simulink model "PT1sys"  (R2016b)
settings: Solver=VariableStepAuto  StartTime=0.0  StopTime=15  RelTol=1e-3
values from neighbouring files (symbols this model uses):
  r1 = 0.0191    [LQG.m]    (also in RiccatiBerechnung_Anlage.m = 0.046; RiccatiBerechnunguPlot_Simulation.m = 0.046; StartSim.m = 0.046)
  T1 = 0.1    [LQG.m]    (also in RiccatiBerechnung_Anlage.m = 0.03032; RiccatiBerechnunguPlot_Simulation.m = 0.03032; StartSim.m = 0.03032)
  T2 = 0.1    [LQG.m]    (also in RiccatiBerechnung_Anlage.m = 0.0247; RiccatiBerechnunguPlot_Simulation.m = 0.0247; StartSim.m = 0.03032)
undefined symbols (not defined in the file or in its folder): K, k1, k2, n01, n02
libraries: simulink x4, simulink_extras x2
settings Model: Creator=Patrick  LastModifiedBy=Patrick

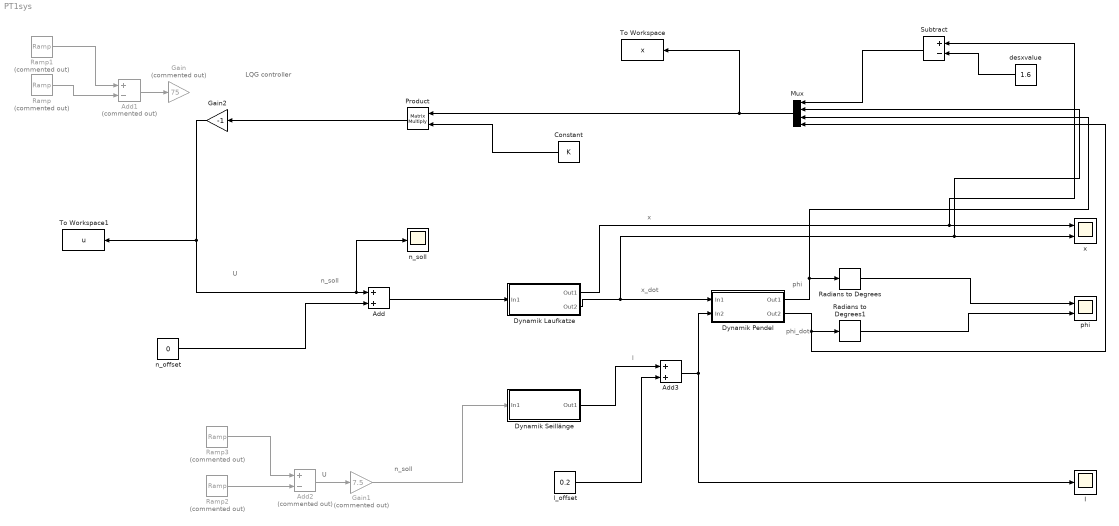
== system PT1sys ==
  note: n_soll
  note: x_dot
  note: U
  note: l
  note: n_soll
  note: U
  note: x
  note: phi
  note: phi_dot
  note: LQG controller
  Add : Sum
  Add1 : Sum  Commented=on  Inputs=+-
  Add2 : Sum  Commented=on  Inputs=+-
  Add3 : Sum
  Constant : Constant  Value=K
  Dynamik Laufkatze : Subsystem
  "Dynamik Pendel " : Subsystem
  Dynamik Seillänge : Subsystem
  Gain : Gain  Commented=on  Gain=75
  Gain1 : Gain  Commented=on  Gain=7.5
  Gain2 : Gain  Gain=-1
  Mux : Mux
  Product : Product  Multiplication=Matrix(*)  SampleTime=0.001  RndMeth=Zero
  Radians to Degrees : simulink_extras/Transformations/Radians to Degrees
  Radians to Degrees1 : simulink_extras/Transformations/Radians to Degrees
  Ramp : simulink/Sources/Ramp  Commented=on  slope=-0.05  start=2  X0=0
  Ramp1 : simulink/Sources/Ramp  Commented=on  slope=-0.05  start=0  X0=0
  Ramp2 : simulink/Sources/Ramp  Commented=on  slope=0.2  start=3  X0=0
  Ramp3 : simulink/Sources/Ramp  Commented=on  slope=0.2  start=0  X0=0
  Subtract : Sum  Inputs=+-
  To Workspace : ToWorkspace  VariableName=x  SampleTime=-1
  To Workspace1 : ToWorkspace  VariableName=u  SampleTime=-1
  desxvalue : Constant  Value=1.6
  l : Scope
  l_offset : Constant  Value=0.2
  n_offset : Constant  Value=0
  n_soll : Scope
  phi : Scope  NumInputPorts=2
  x : Scope  NumInputPorts=2
  wires:
  n_offset/1 -> Add/2
  Dynamik Laufkatze/2(Out2) -> "Dynamik Pendel "/1(In1), x/2, Mux/2
  Gain2/1 -> n_soll/1, Add/1, To Workspace1/1
  Ramp1/1 -> Add1/1
  Ramp/1 -> Add1/2
  Ramp3/1 -> Add2/1
  Add2/1 -> Gain1/1
  Ramp2/1 -> Add2/2
  Gain1/1 -> Dynamik Seillänge/1(In1)
  Dynamik Seillänge/1(Out1) -> Add3/1
  l_offset/1 -> Add3/2
  Add3/1 -> l/1, "Dynamik Pendel "/2(In2)
  "Dynamik Pendel "/1(Out1) -> Mux/3, Radians to Degrees/1
  Radians to Degrees/1 -> phi/1
  "Dynamik Pendel "/2(Out2) -> Mux/4, Radians to Degrees1/1
  Radians to Degrees1/1 -> phi/2
  Product/1 -> Gain2/1
  Constant/1 -> Product/2
  Dynamik Laufkatze/1(Out1) -> Subtract/1, x/1
  Mux/1 -> To Workspace/1, Product/1
  Add/1 -> Dynamik Laufkatze/1(In1)
  desxvalue/1 -> Subtract/2
  Subtract/1 -> Mux/1
  Add1/1 -> Gain/1

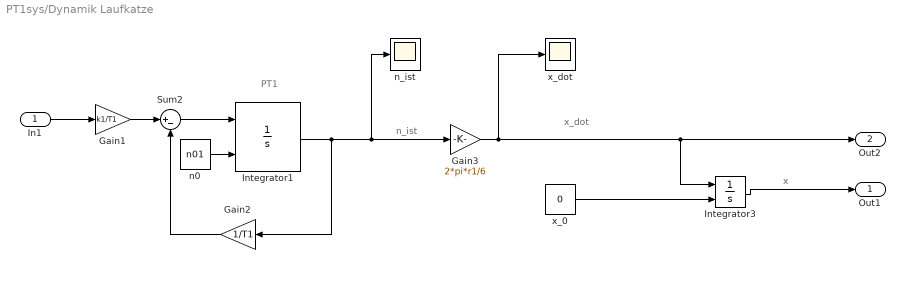
== system PT1sys/Dynamik Laufkatze ==
  note: n_ist
  note: PT1
  note: x_dot
  note: x
  In1 : Inport
  Gain1 : Gain  Gain=k1/T1
  Gain2 : Gain  Gain=1/T1
  Gain3 : Gain  Gain=2*pi*r1/6
  Integrator1 : Integrator  InitialConditionSource=external
  Integrator3 : Integrator  InitialConditionSource=external
  Sum2 : Sum  Inputs=|+-
  n0 : Constant  Value=n01
  n_ist : Scope
  x_0 : Constant  Value=0
  x_dot : Scope
  Out1 : Outport
  Out2 : Outport  Port=2
  wires:
  Gain3/1 -> Out2/1, Integrator3/1, x_dot/1
  Sum2/1 -> Integrator1/1
  Gain2/1 -> Sum2/2
  Integrator1/1 -> n_ist/1, Gain3/1, Gain2/1
  Gain1/1 -> Sum2/1
  In1/1 -> Gain1/1
  Integrator3/1 -> Out1/1
  n0/1 -> Integrator1/2
  x_0/1 -> Integrator3/2

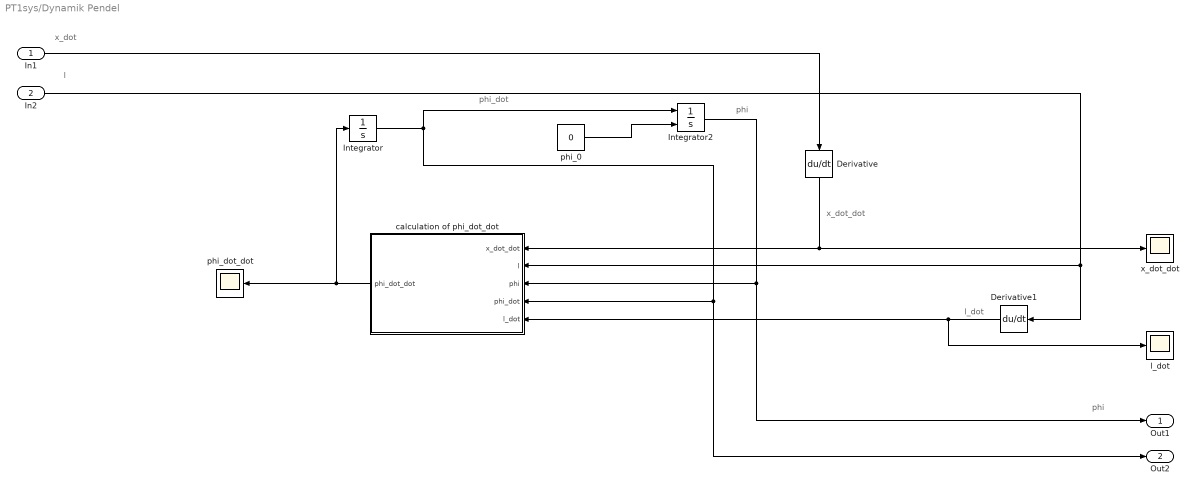
== system PT1sys/Dynamik Pendel  ==
  note: x_dot_dot
  note: phi_dot
  note: phi
  note: x_dot
  note: l
  note: phi
  note: l_dot
  In1 : Inport
  In2 : Inport  Port=2
  Derivative : Derivative
  Derivative1 : Derivative
  Integrator : Integrator
  Integrator2 : Integrator  InitialConditionSource=external
  calculation of phi_dot_dot : MATLAB Function  TreatAsAtomicUnit=on
  l_dot : Scope
  phi_0 : Constant  Value=0
  phi_dot_dot : Scope
  x_dot_dot : Scope
  Out1 : Outport
  Out2 : Outport  Port=2
  wires:
  Derivative/1 -> calculation of phi_dot_dot/1(x_dot_dot), x_dot_dot/1
  Integrator2/1 -> calculation of phi_dot_dot/3(phi), Out1/1
  calculation of phi_dot_dot/1(phi_dot_dot) -> Integrator/1, phi_dot_dot/1
  Integrator/1 -> Out2/1, calculation of phi_dot_dot/4(phi_dot), Integrator2/1
  In1/1 -> Derivative/1
  In2/1 -> Derivative1/1, calculation of phi_dot_dot/2(l)
  Derivative1/1 -> l_dot/1, calculation of phi_dot_dot/5(l_dot)
  phi_0/1 -> Integrator2/2

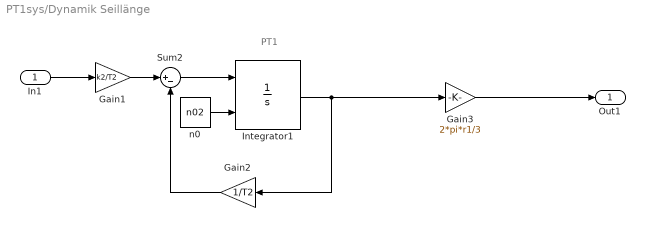
== system PT1sys/Dynamik Seillänge ==
  note: PT1
  In1 : Inport
  Gain1 : Gain  Gain=k2/T2
  Gain2 : Gain  Gain=1/T2
  Gain3 : Gain  Gain=2*pi*r1/3
  Integrator1 : Integrator  InitialConditionSource=external
  Sum2 : Sum  Inputs=|+-
  n0 : Constant  Value=n02
  Out1 : Outport
  wires:
  n0/1 -> Integrator1/2
  Sum2/1 -> Integrator1/1
  Gain2/1 -> Sum2/2
  Integrator1/1 -> Gain3/1, Gain2/1
  Gain1/1 -> Sum2/1
  In1/1 -> Gain1/1
  Gain3/1 -> Out1/1

== matlab function PT1sys/Dynamik Pendel /calculation of phi_dot_dot ==
  data: x_dot_dot input; phi_dot_dot output; l input; phi input; phi_dot input; l_dot input
function phi_dot_dot = fcn(x_dot_dot,l,phi,phi_dot,l_dot)

phi_dot_dot = -(cos(phi)/l)*x_dot_dot-9.81/l*sin(phi)+2*l_dot*phi_dot;
